simulink model "mathSimulink"  (R2017a)
settings: Solver=VariableStepAuto  StartTime=0.0  StopTime=10.0  RelTol=1e-3
settings Model: Creator=Pc  LastModifiedBy=Pc

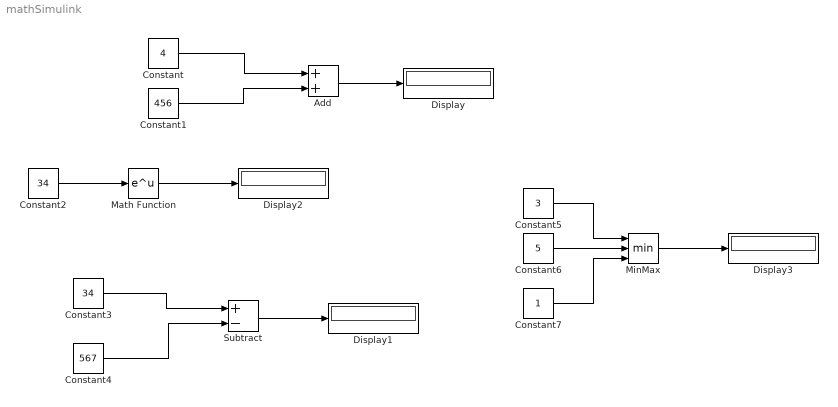
== system mathSimulink ==
  Add : Sum
  Constant : Constant  Value=4
  Constant1 : Constant  Value=456
  Constant2 : Constant  Value=34
  Constant3 : Constant  Value=34
  Constant4 : Constant  Value=567
  Constant5 : Constant  Value=3
  Constant6 : Constant  Value=5
  Constant7 : Constant
  Display{,1..3} (4 alike) : Display
  Math Function : Math  SaturateOnIntegerOverflow=on
  MinMax : MinMax  Inputs=3
  Subtract : Sum  Inputs=+-
  wires:
  Constant/1 -> Add/1
  Constant1/1 -> Add/2
  Add/1 -> Display/1
  Constant2/1 -> Math Function/1
  Math Function/1 -> Display2/1
  Constant3/1 -> Subtract/1
  Constant4/1 -> Subtract/2
  Subtract/1 -> Display1/1
  Constant5/1 -> MinMax/1
  MinMax/1 -> Display3/1
  Constant6/1 -> MinMax/2
  Constant7/1 -> MinMax/3
